simulink model "Thermal_cooling_sim"  (R2025b)
settings: Solver=ode15s  StartTime=0  StopTime=25  MaxStep=1e-2  MinStep=1e-6  RelTol=1e-2  AbsTol=1e-6  EnableMultiTasking=on
PreLoadFcn:
  | PMSMDriveThermalData;
libraries: batteryecm_lib x281, fl_lib x58, nesl_utility x25, ee_lib x9, SimscapeFluids_lib x3, eePmsmFieldOrientedControl x1, BatteryEstimators x1
(part 24 of 24)

== system Thermal_cooling_sim/Cooling system/Subsystem1 ==
  Inverter Power_loss : Scope
      settings: ActiveDisplayYMinimum=308.1365205491262  ActiveDisplayYMaximum=1104.1464495560401  DataLoggingVariableName=ScopeData3
  PS Lookup Table (2D) : fl_lib/Physical Signals/Lookup Tables/PS Lookup Table (2D)  x1=[100, 150, 200, 250, 300, 350, 400, 450, 500, 550, 600, 650, 700, 750, 800] V  x2=[100, 150, 200, 250, 300, 350, 400, 450, 500, 550, 600] A  f=|  interp_method=simscape.enum.interpolation.smooth  extrap_method=simscape.enum.extrapolation.nearest
      | [199.5, 318, 436.5, 580.5, 724.5, 899.8, 1075, 1267.5, 1460, 1692.5, 1925;
      | 230.3, 362.3, 494.3, 651.8, 809.3, 998.4, 1187.5, 1393.8, 1600, 1843.8, 2087.5;
      | 261, 406.5, 552, 723, 894, 1097, 1300, 1520, 1740, 1995, 2250;
      | 291.8, 450.8, 609.8, 794.3, 978.8, 1195.6, 1412.5, 1646.3, 1880, 2146.3, 2412.5;
      | 322.5, 495, 667.5, 865.5, 1063.5, 1294.3, 1525, 1772.5, 2020, 2297.5, 2575;
      | 353.3, 539.3, 725.3, 936.8, 1148.3, 1392.9, 1637.5, 1898.8, 2160, 2448.8, 2737.5;
      | 384, 583.5, 783, 1008, 1233, 1491.5, 1750, 2025, 2300, 2600, 2900;
      | 416.3, 629.3, 842.3, 1081.5, 1320.8, 1591.6, 1862.5, 2156.3, 2450, 2768.8, 3087.5;
      | 448.5, 675, 901.5, 1155, 1408.5, 1691.8, 1975, 2287.5, 2600, 2937.5, 3275;
      | 480.8, 720.8, 960.8, 1228.5, 1496.3, 1791.9, 2087.5, 2418.8, 2750, 3106.3, 3462.5;
      | 513, 766.5, 1020, 1302, 1584, 1892, 2200, 2550, 2900, 3275, 3650;
      | 545.3, 812.6, 1080, 1378.5, 1677, 2006, 2335, 2698.8, 3062.5, 3462.5, 3862.5;
      | 577.5, 858.8, 1140, 1455, 1770, 2120, 2470, 2847.5, 3225, 3650, 4075;
      | 609.8, 904.9, 1200, 1531.5, 1863, 2234, 2605, 2996.3, 3387.5, 3837.5, 4287.5;
      | 642, 951, 1260, 1608, 1956, 2348, 2740, 3145, 3550, 4025, 4500] W
  PS-Simulink Converter : nesl_utility/PS-Simulink Converter  PhysicalDomain=network_engine_domain  SubClassName=ps_output  LeftPortType=input  RightPortType=output  PseudoPeriodic=off  Frequencies=[]  VectorFormat=inherit  Unit=W  AffineConversion=off
  ARMS_IN : PMIOPort  Side=Left
  VDC_IN : PMIOPort  Port=2  Side=Left
  output : PMIOPort  Port=3  Side=Right
  wires:
  PS-Simulink Converter/1 -> Inverter Power_loss/1
  connections:
  PS-Simulink Converter/LConn1 -- output/RConn1 -- PS Lookup Table (2D)/RConn1
  PS Lookup Table (2D)/LConn1 -- VDC_IN/RConn1
  PS Lookup Table (2D)/LConn2 -- ARMS_IN/RConn1

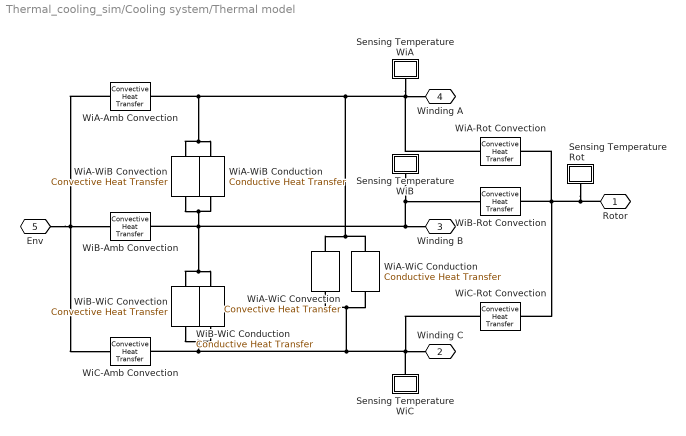
== system Thermal_cooling_sim/Cooling system/Thermal model ==
  Sensing Temperature Rot : Subsystem
      mask Display: disp('TR')
  Sensing Temperature WiA : Subsystem
      mask Display: disp('TA')
  Sensing Temperature WiB : Subsystem
      mask Display: disp('TB')
  Sensing Temperature WiC : Subsystem
      mask Display: disp('TC')
  WiA-Amb Convection : fl_lib/Thermal/Thermal Elements/Convective Heat Transfer  thermal_type=foundation.enum.constant_variable.constant  area=0.1 m^2  heat_tr_coeff=20 W/(m^2 * K)  min_heat_tr_coeff=1e-3 W/(K*m^2)  T_specify=off  T_priority=None  T=0 K  T_nominal_specify=off  T_nominal_value=1  T_nominal_unit=K  Q_specify=off  Q_priority=None  Q=0 J/s  Q_nominal_specify=off  Q_nominal_value=1  Q_nominal_unit=J/s
  WiA-Rot Convection : fl_lib/Thermal/Thermal Elements/Convective Heat Transfer  thermal_type=foundation.enum.constant_variable.constant  area=0.02 m^2  heat_tr_coeff=200 W/(m^2 * K)  min_heat_tr_coeff=1e-3 W/(K*m^2)  T_specify=off  T_priority=None  T=0 K  T_nominal_specify=off  T_nominal_value=1  T_nominal_unit=K  Q_specify=off  Q_priority=None  Q=0 J/s  Q_nominal_specify=off  Q_nominal_value=1  Q_nominal_unit=J/s
  WiA-WiB Conduction : fl_lib/Thermal/Thermal Elements/Conductive Heat Transfer  thermal_type=foundation.enum.ConstantVariableTabulated.Constant  wall_geometry=foundation.enum.ConductionWallGeometry.Planar  area=0.002 m^2  thickness=0.1 m  d_in=0.05 m  d_out=0.1 m  L=1 m  th_cond_min=10 W/(K*m)  th_cond=80 W/(m*K)  th_cond_TLU=[413, 401, 392, 383, 371, 357, 342] W/(K*m)  temp_TLU=[200, 273, 400, 600, 800, 1000, 1200] K  T_specify=off  T_priority=None  T=0 K  T_nominal_specify=off  T_nominal_value=1  T_nominal_unit=K  Q_specify=off  Q_priority=None  Q=0 J/s  Q_nominal_specify=off  Q_nominal_value=1  Q_nominal_unit=J/s
  WiA-WiB Convection : fl_lib/Thermal/Thermal Elements/Convective Heat Transfer  thermal_type=foundation.enum.constant_variable.constant  area=0.004 m^2  heat_tr_coeff=200 W/(m^2 * K)  min_heat_tr_coeff=1e-3 W/(K*m^2)  T_specify=off  T_priority=None  T=0 K  T_nominal_specify=off  T_nominal_value=1  T_nominal_unit=K  Q_specify=off  Q_priority=None  Q=0 J/s  Q_nominal_specify=off  Q_nominal_value=1  Q_nominal_unit=J/s
  WiA-WiC Conduction : fl_lib/Thermal/Thermal Elements/Conductive Heat Transfer  thermal_type=foundation.enum.ConstantVariableTabulated.Constant  wall_geometry=foundation.enum.ConductionWallGeometry.Planar  area=0.002 m^2  thickness=0.1 m  d_in=0.05 m  d_out=0.1 m  L=1 m  th_cond_min=10 W/(K*m)  th_cond=80 W/(m*K)  th_cond_TLU=[413, 401, 392, 383, 371, 357, 342] W/(K*m)  temp_TLU=[200, 273, 400, 600, 800, 1000, 1200] K  T_specify=off  T_priority=None  T=0 K  T_nominal_specify=off  T_nominal_value=1  T_nominal_unit=K  Q_specify=off  Q_priority=None  Q=0 J/s  Q_nominal_specify=off  Q_nominal_value=1  Q_nominal_unit=J/s
  WiA-WiC Convection : fl_lib/Thermal/Thermal Elements/Convective Heat Transfer  thermal_type=foundation.enum.constant_variable.constant  area=0.004 m^2  heat_tr_coeff=200 W/(m^2 * K)  min_heat_tr_coeff=1e-3 W/(K*m^2)  T_specify=off  T_priority=None  T=0 K  T_nominal_specify=off  T_nominal_value=1  T_nominal_unit=K  Q_specify=off  Q_priority=None  Q=0 J/s  Q_nominal_specify=off  Q_nominal_value=1  Q_nominal_unit=J/s
  WiB-Amb Convection : fl_lib/Thermal/Thermal Elements/Convective Heat Transfer  thermal_type=foundation.enum.constant_variable.constant  area=0.1 m^2  heat_tr_coeff=20 W/(m^2 * K)  min_heat_tr_coeff=1e-3 W/(K*m^2)  T_specify=off  T_priority=None  T=0 K  T_nominal_specify=off  T_nominal_value=1  T_nominal_unit=K  Q_specify=off  Q_priority=None  Q=0 J/s  Q_nominal_specify=off  Q_nominal_value=1  Q_nominal_unit=J/s
  WiB-Rot Convection : fl_lib/Thermal/Thermal Elements/Convective Heat Transfer  thermal_type=foundation.enum.constant_variable.constant  area=0.02 m^2  heat_tr_coeff=200 W/(m^2 * K)  min_heat_tr_coeff=1e-3 W/(K*m^2)  T_specify=off  T_priority=None  T=0 K  T_nominal_specify=off  T_nominal_value=1  T_nominal_unit=K  Q_specify=off  Q_priority=None  Q=0 J/s  Q_nominal_specify=off  Q_nominal_value=1  Q_nominal_unit=J/s
  WiB-WiC Conduction : fl_lib/Thermal/Thermal Elements/Conductive Heat Transfer  thermal_type=foundation.enum.ConstantVariableTabulated.Constant  wall_geometry=foundation.enum.ConductionWallGeometry.Planar  area=0.002 m^2  thickness=0.1 m  d_in=0.05 m  d_out=0.1 m  L=1 m  th_cond_min=10 W/(K*m)  th_cond=80 W/(m*K)  th_cond_TLU=[413, 401, 392, 383, 371, 357, 342] W/(K*m)  temp_TLU=[200, 273, 400, 600, 800, 1000, 1200] K  T_specify=off  T_priority=None  T=0 K  T_nominal_specify=off  T_nominal_value=1  T_nominal_unit=K  Q_specify=off  Q_priority=None  Q=0 J/s  Q_nominal_specify=off  Q_nominal_value=1  Q_nominal_unit=J/s
  WiB-WiC Convection : fl_lib/Thermal/Thermal Elements/Convective Heat Transfer  thermal_type=foundation.enum.constant_variable.constant  area=0.004 m^2  heat_tr_coeff=200 W/(m^2 * K)  min_heat_tr_coeff=1e-3 W/(K*m^2)  T_specify=off  T_priority=None  T=0 K  T_nominal_specify=off  T_nominal_value=1  T_nominal_unit=K  Q_specify=off  Q_priority=None  Q=0 J/s  Q_nominal_specify=off  Q_nominal_value=1  Q_nominal_unit=J/s
  WiC-Amb Convection : fl_lib/Thermal/Thermal Elements/Convective Heat Transfer  thermal_type=foundation.enum.constant_variable.constant  area=0.1 m^2  heat_tr_coeff=20 W/(m^2 * K)  min_heat_tr_coeff=1e-3 W/(K*m^2)  T_specify=off  T_priority=None  T=0 K  T_nominal_specify=off  T_nominal_value=1  T_nominal_unit=K  Q_specify=off  Q_priority=None  Q=0 J/s  Q_nominal_specify=off  Q_nominal_value=1  Q_nominal_unit=J/s
  WiC-Rot Convection : fl_lib/Thermal/Thermal Elements/Convective Heat Transfer  thermal_type=foundation.enum.constant_variable.constant  area=0.02 m^2  heat_tr_coeff=200 W/(m^2 * K)  min_heat_tr_coeff=1e-3 W/(K*m^2)  T_specify=off  T_priority=None  T=0 K  T_nominal_specify=off  T_nominal_value=1  T_nominal_unit=K  Q_specify=off  Q_priority=None  Q=0 J/s  Q_nominal_specify=off  Q_nominal_value=1  Q_nominal_unit=J/s
  Rotor : PMIOPort  Side=Left
  Winding C : PMIOPort  Port=2  Side=Right
  Winding B : PMIOPort  Port=3  Side=Right
  Winding A : PMIOPort  Port=4  Side=Right
  Env : PMIOPort  Port=5  Side=Left
  connections:
  WiA-Rot Convection/RConn1 -- WiA-WiC Conduction/RConn1 -- WiA-WiC Convection/RConn1 -- WiA-WiB Convection/LConn1 -- WiA-WiB Conduction/LConn1 -- WiA-Amb Convection/LConn1 -- Sensing Temperature WiA/LConn1 -- Winding A/RConn1
  Rotor/RConn1 -- Sensing Temperature Rot/LConn1 -- WiC-Rot Convection/LConn1 -- WiB-Rot Convection/LConn1 -- WiA-Rot Convection/LConn1
  WiA-WiB Convection/RConn1 -- WiA-WiB Conduction/RConn1 -- Sensing Temperature WiB/LConn1 -- WiB-Rot Convection/RConn1 -- Winding B/RConn1 -- WiB-Amb Convection/LConn1 -- WiB-WiC Conduction/LConn1 -- WiB-WiC Convection/LConn1
  WiC-Rot Convection/RConn1 -- Winding C/RConn1 -- WiB-WiC Conduction/RConn1 -- WiB-WiC Convection/RConn1 -- WiC-Amb Convection/LConn1 -- WiA-WiC Convection/LConn1 -- WiA-WiC Conduction/LConn1 -- Sensing Temperature WiC/LConn1
  WiA-Amb Convection/RConn1 -- Env/RConn1 -- WiC-Amb Convection/RConn1 -- WiB-Amb Convection/RConn1

== system Thermal_cooling_sim/Throttle controller/ Torque Reference ==
  Throtte Positon : Inport  Unit=km/hr
  Constant : Constant  Value=240
  Divide : Product  Inputs=*/
  From Workspace : FromWorkspace  Commented=on  VariableName=Current_Matrix
  Gain : Gain  Gain=0.57735026919
  Gain1 : Gain  Gain=0.83
  Product : Product
  Torque ref : Scope
      settings: ActiveDisplayYMinimum=-13.959117073448896  ActiveDisplayYMaximum=125.63205366104009  DataLoggingVariableName=ScopeData11
  percentage : Constant  Value=100
  Motortrqref : Outport  Unit=rpm  VectorParamsAs1DForOutWhenUnconnected=off
  wires:
  Throtte Positon/1 -> Divide/1
  percentage/1 -> Divide/2
  Divide/1 -> Product/2
  Constant/1 -> Product/1
  Product/1 -> Gain/1
  Gain/1 -> Gain1/1
  Gain1/1 -> Torque ref/1, Motortrqref/1

== system Thermal_cooling_sim/Throttle controller/Control ==
  note: Is Pressure an output?
  Torque Ref : Inport
  motorspd : Inport  Port=2
  bus voltage : Inport  Port=3
  SOC : Inport  Port=4
  20Hz Lowpass Filter : TransferFcn  Denominator=[1/(2*pi*20) 1]
  Cmd Torque : Scope
      settings: ActiveDisplayYMinimum=-13.959117072781753  ActiveDisplayYMaximum=125.6320536550358
  Motor Torque : Subsystem
  MotCmdTrq : Outport
  wires:
  Motor Torque/1(motTrq) -> 20Hz Lowpass Filter/1  "MotCmdTrq"
  SOC/1 -> Motor Torque/2(SOC)
  bus voltage/1 -> Motor Torque/3(bus voltage)
  motorspd/1 -> Motor Torque/4(motorspd)
  Torque Ref/1 -> Motor Torque/1(trqReq)
  20Hz Lowpass Filter/1 -> Cmd Torque/1, MotCmdTrq/1  "Motor Speed"

== system Thermal_cooling_sim/Cooling system/Cooling system /Sensing Temperature Inverter ==
  PS-Simulink Converter : nesl_utility/PS-Simulink Converter  PhysicalDomain=network_engine_domain  SubClassName=ps_output  LeftPortType=input  RightPortType=output  PseudoPeriodic=off  Frequencies=[]  VectorFormat=1-D array  Unit=degC  AffineConversion=on
  Temperature Sensor : fl_lib/Thermal/Thermal Sensors/Temperature Sensor  temperature_measure=foundation.enum.MeasurementReference.difference
  ThRef : fl_lib/Thermal/Thermal Elements/Thermal Reference
  H : PMIOPort  Side=Left
  Cooling Inverter : Outport
  wires:
  PS-Simulink Converter/1 -> Cooling Inverter/1
  connections:
  ThRef/LConn1 -- Temperature Sensor/RConn1
  H/RConn1 -- Temperature Sensor/LConn1
  Temperature Sensor/RConn2 -- PS-Simulink Converter/LConn1

== system Thermal_cooling_sim/Cooling system/Cooling system /Sensing Temperature Inverter1 ==
  PS-Simulink Converter : nesl_utility/PS-Simulink Converter  PhysicalDomain=network_engine_domain  SubClassName=ps_output  LeftPortType=input  RightPortType=output  PseudoPeriodic=off  Frequencies=[]  VectorFormat=1-D array  Unit=degC  AffineConversion=on
  Temperature Sensor : fl_lib/Thermal/Thermal Sensors/Temperature Sensor  temperature_measure=foundation.enum.MeasurementReference.difference
  ThRef : fl_lib/Thermal/Thermal Elements/Thermal Reference
  H : PMIOPort  Side=Left
  Cooling motor : Outport
  wires:
  PS-Simulink Converter/1 -> Cooling motor/1
  connections:
  ThRef/LConn1 -- Temperature Sensor/RConn1
  H/RConn1 -- Temperature Sensor/LConn1
  Temperature Sensor/RConn2 -- PS-Simulink Converter/LConn1

== system Thermal_cooling_sim/Cooling system/Cooling system /Subsystem ==
  "Motor Temp " : Scope
      settings: ActiveDisplayYMinimum=24.711691624047347  ActiveDisplayYMaximum=27.2437474538107  DataLoggingVariableName=ScopeData2
  PS-Simulink Converter : nesl_utility/PS-Simulink Converter  PhysicalDomain=network_engine_domain  SubClassName=ps_output  LeftPortType=input  RightPortType=output  PseudoPeriodic=off  Frequencies=[]  VectorFormat=inherit  Unit=degC  AffineConversion=on
  Temperature Sensor : fl_lib/Thermal/Thermal Sensors/Temperature Sensor  temperature_measure=foundation.enum.MeasurementReference.difference
  Thermal Reference : fl_lib/Thermal/Thermal Elements/Thermal Reference
  Conn1 : PMIOPort  Side=Left
  wires:
  PS-Simulink Converter/1 -> "Motor Temp "/1  "Motor Temperature"
  connections:
  Temperature Sensor/LConn1 -- Conn1/RConn1
  Thermal Reference/LConn1 -- Temperature Sensor/RConn1
  PS-Simulink Converter/LConn1 -- Temperature Sensor/RConn2

== system Thermal_cooling_sim/Cooling system/Thermal model/Sensing Temperature Rot ==
  PS-Simulink Converter : nesl_utility/PS-Simulink Converter  PhysicalDomain=network_engine_domain  SubClassName=ps_output  LeftPortType=input  RightPortType=output  PseudoPeriodic=off  Frequencies=[]  VectorFormat=1-D array  Unit=degC  AffineConversion=on
  Temperature Sensor : fl_lib/Thermal/Thermal Sensors/Temperature Sensor  temperature_measure=foundation.enum.MeasurementReference.difference
  ThRef : fl_lib/Thermal/Thermal Elements/Thermal Reference
  H : PMIOPort  Side=Left
  tag scope: TR=global
  wires:
  PS-Simulink Converter/1 -> [TR]
  connections:
  Temperature Sensor/RConn2 -- PS-Simulink Converter/LConn1
  ThRef/LConn1 -- Temperature Sensor/RConn1
  H/RConn1 -- Temperature Sensor/LConn1

== system Thermal_cooling_sim/Cooling system/Thermal model/Sensing Temperature WiA ==
  PS-Simulink Converter : nesl_utility/PS-Simulink Converter  PhysicalDomain=network_engine_domain  SubClassName=ps_output  LeftPortType=input  RightPortType=output  PseudoPeriodic=off  Frequencies=[]  VectorFormat=1-D array  Unit=degC  AffineConversion=on
  Temperature Sensor : fl_lib/Thermal/Thermal Sensors/Temperature Sensor  temperature_measure=foundation.enum.MeasurementReference.difference
  ThRef : fl_lib/Thermal/Thermal Elements/Thermal Reference
  H : PMIOPort  Side=Left
  tag scope: TA=global
  wires:
  PS-Simulink Converter/1 -> [TA]
  connections:
  H/RConn1 -- Temperature Sensor/LConn1
  ThRef/LConn1 -- Temperature Sensor/RConn1
  Temperature Sensor/RConn2 -- PS-Simulink Converter/LConn1

== system Thermal_cooling_sim/Cooling system/Thermal model/Sensing Temperature WiB ==
  PS-Simulink Converter : nesl_utility/PS-Simulink Converter  PhysicalDomain=network_engine_domain  SubClassName=ps_output  LeftPortType=input  RightPortType=output  PseudoPeriodic=off  Frequencies=[]  VectorFormat=1-D array  Unit=degC  AffineConversion=on
  Temperature Sensor : fl_lib/Thermal/Thermal Sensors/Temperature Sensor  temperature_measure=foundation.enum.MeasurementReference.difference
  ThRef : fl_lib/Thermal/Thermal Elements/Thermal Reference
  H : PMIOPort  Side=Left
  tag scope: TB=global
  wires:
  PS-Simulink Converter/1 -> [TB]
  connections:
  ThRef/LConn1 -- Temperature Sensor/RConn1
  H/RConn1 -- Temperature Sensor/LConn1
  Temperature Sensor/RConn2 -- PS-Simulink Converter/LConn1

== system Thermal_cooling_sim/Cooling system/Thermal model/Sensing Temperature WiC ==
  PS-Simulink Converter : nesl_utility/PS-Simulink Converter  PhysicalDomain=network_engine_domain  SubClassName=ps_output  LeftPortType=input  RightPortType=output  PseudoPeriodic=off  Frequencies=[]  VectorFormat=1-D array  Unit=degC  AffineConversion=on
  Temperature Sensor : fl_lib/Thermal/Thermal Sensors/Temperature Sensor  temperature_measure=foundation.enum.MeasurementReference.difference
  ThRef : fl_lib/Thermal/Thermal Elements/Thermal Reference
  H : PMIOPort  Side=Left
  tag scope: TC=global
  wires:
  PS-Simulink Converter/1 -> [TC]
  connections:
  H/RConn1 -- Temperature Sensor/LConn1
  ThRef/LConn1 -- Temperature Sensor/RConn1
  Temperature Sensor/RConn2 -- PS-Simulink Converter/LConn1

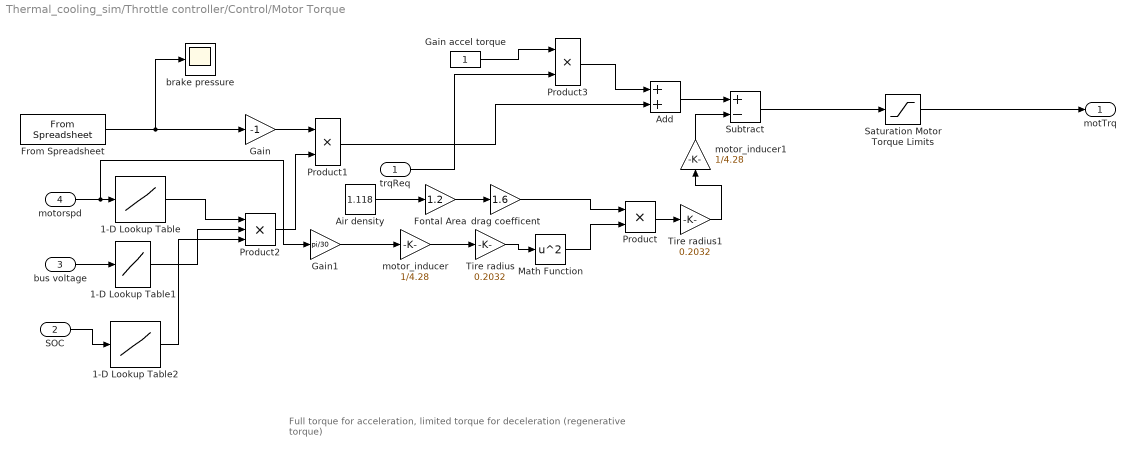
== system Thermal_cooling_sim/Throttle controller/Control/Motor Torque ==
  note: Full torque for acceleration,
      | limited torque for deceleration (regenerative torque)
  trqReq : Inport
  SOC : Inport  Port=2
  bus voltage : Inport  Port=3
  motorspd : Inport  Port=4
  1-D Lookup Table : Lookup_n-D  NumberOfTableDimensions=1  BreakpointsForDimension1=[0,8,15,999]  Table=[0,0,1,1]  InternalRulePriority=Speed  RndMeth=Simplest
  1-D Lookup Table1 : Lookup_n-D  NumberOfTableDimensions=1  BreakpointsForDimension1=[0,540,560,999]  Table=[1,1,0,0]  InternalRulePriority=Speed  RndMeth=Simplest
  1-D Lookup Table2 : Lookup_n-D  NumberOfTableDimensions=1  BreakpointsForDimension1=[0,0.8,0.95,1]  Table=[1,1,0,0]  InternalRulePriority=Speed  RndMeth=Simplest
  Add : Sum
  Air density : Constant  Value=1.118
  Fontal Area : Gain  Gain=1.2
  From Spreadsheet : FromSpreadsheet  FileName=/Users/muizz_1/Documents/E27-Tractive-system-MATLAB-model-/Models/E25_Run1.xls  SheetName=Brake
  Gain : Gain  Gain=-1
  Gain accel torque : Constant
  Gain1 : Gain  Gain=pi/30
  Math Function : Math  Operator=square
  Product : Product
  Product1 : Product
  Product2 : Product  Inputs=3
  Product3 : Product
  Saturation Motor Torque Limits : Saturate  UpperLimit=150  LowerLimit=-150  ZeroCross=off
  Subtract : Sum  Inputs=+-
  Tire radius : Gain  Gain=0.2032
  Tire radius1 : Gain  Gain=0.2032
  brake pressure : Scope
      settings: ActiveDisplayYMinimum=-30.006488969158148  ActiveDisplayYMaximum=54.0625428368765  DataLoggingVariableName=ScopeData10
  drag coefficent : Gain  Gain=1.6
  motor_inducer : Gain  Gain=1/4.28
  motor_inducer1 : Gain  Gain=1/4.28
  motTrq : Outport
  wires:
  Saturation Motor Torque Limits/1 -> motTrq/1
  From Spreadsheet/1 -> brake pressure/1, Gain/1
  Gain/1 -> Product1/1
  SOC/1 -> 1-D Lookup Table2/1
  bus voltage/1 -> 1-D Lookup Table1/1
  1-D Lookup Table/1 -> Product2/1
  1-D Lookup Table1/1 -> Product2/2
  1-D Lookup Table2/1 -> Product2/3
  Product2/1 -> Product1/2
  Product1/1 -> Add/2
  Gain accel torque/1 -> Product3/1
  trqReq/1 -> Product3/2
  Product3/1 -> Add/1
  Add/1 -> Subtract/1
  Subtract/1 -> Saturation Motor Torque Limits/1
  Air density/1 -> Fontal Area/1
  Fontal Area/1 -> drag coefficent/1
  motorspd/1 -> Gain1/1, 1-D Lookup Table/1
  motor_inducer/1 -> Tire radius/1
  Tire radius/1 -> Math Function/1
  Math Function/1 -> Product/2
  drag coefficent/1 -> Product/1
  Tire radius1/1 -> motor_inducer1/1
  Product/1 -> Tire radius1/1
  motor_inducer1/1 -> Subtract/2
  Gain1/1 -> motor_inducer/1
